simulink model "testbench_main2"  (R2016b)
settings: Solver=FixedStepAuto  StartTime=0.0  StopTime=inf  RelTol=1e-3  EnableMultiTasking=on
values from neighbouring files (symbols this model uses):
  b = 16    [Script_controller.m]
libraries: legoev3lib x4
settings Model: SimulationMode=external  ExtModeTrigDuration=2  Creator=Shobhit  LastModifiedBy=karanverma
settings SolverCC: PositivePriorityOrder=on
settings OptimizationCC: LifeSpan=1  MaxStackSize=64
settings DebuggingCC: SFUnexpectedBacktrackingDiag=warning  SFNoUnconditionalDefaultTransitionDiag=warning  SFExecutionAtInitializationDiag=none
settings HardwareCC: ProdBitPerPointer=32  ProdBitPerSizeT=32  ProdBitPerPtrDiffT=32  ProdLargestAtomicInteger=Long  ProdWordSize=32  ProdHWDeviceType=ARM Compatible->ARM 9  UseEmbeddedCoderFeatures=off  UseSimulinkCoderFeatures=off
settings RTWCC: SystemTargetFile=ert.tlc  HardwareBoard=LEGO MINDSTORMS EV3  TLCOptions=-aInlineSetEventsForThisBaseRateFcn=TLC_FALSE -aSuppressMultiTaskScheduler=TLC_FALSE -aRateBasedStepFcn=0  TemplateMakefile=ert_default_tmf  Description=Embedded Coder  GenerateReport=on  Toolchain=Sourcery G++ Lite v2009q3  LaunchReport=on
settings CodeAppCC: ForceParamTrailComments=on  OperatorAnnotations=on  MATLABSourceComments=on
settings ERTTargetCC: ERTCustomFileBanners=off  SupportContinuousTime=on  SupportNonInlinedSFcns=on  SupportVariableSizeSignals=on  ModelStepFunctionPrototypeControlCompliant=off
settings ConfigComp: CovMetricSettings=dw  CovHtmlReporting=on  CovSaveCumulativeToWorkspaceVar=on  CovSaveSingleToWorkspaceVar=on  CovExternalEMLEnable=off

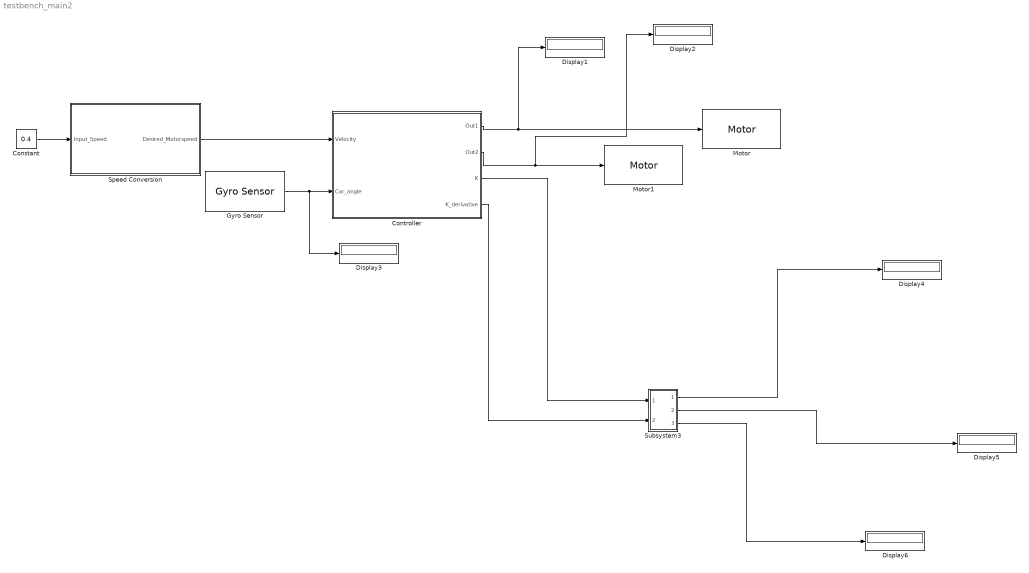
== system testbench_main2 ==
  Constant : Constant  Value=0.4
  Controller : Subsystem
  Display{1..6} (6 alike) : Display
      Display4 settings: Decimation=2
  Gyro Sensor : legoev3lib/Gyro Sensor  portNumber=1  sampleTime=0.1
  Motor : legoev3lib/Motor  sportNumber=A  sstopAction=Brake
  Motor1 : legoev3lib/Motor  sportNumber=B  sstopAction=Brake
  Speed Conversion : Subsystem
  Subsystem3 : Subsystem
  wires:
  Gyro Sensor/1 -> Display3/1, Controller/2(Car_angle)
  Constant/1 -> Speed Conversion/1(Input_Speed)
  Controller/1(Out1) -> Motor/1, Display1/1
  Controller/2(Out2) -> Display2/1, Motor1/1
  Speed Conversion/1(Desired_Motorspeed) -> Controller/1(Velocity)
  Controller/4(K_derivative) -> Subsystem3/2(In2)
  Subsystem3/1(Out1) -> Display4/1
  Subsystem3/2(Out2) -> Display5/1
  Subsystem3/3(Out3) -> Display6/1
  Controller/3(K) -> Subsystem3/1(In1)

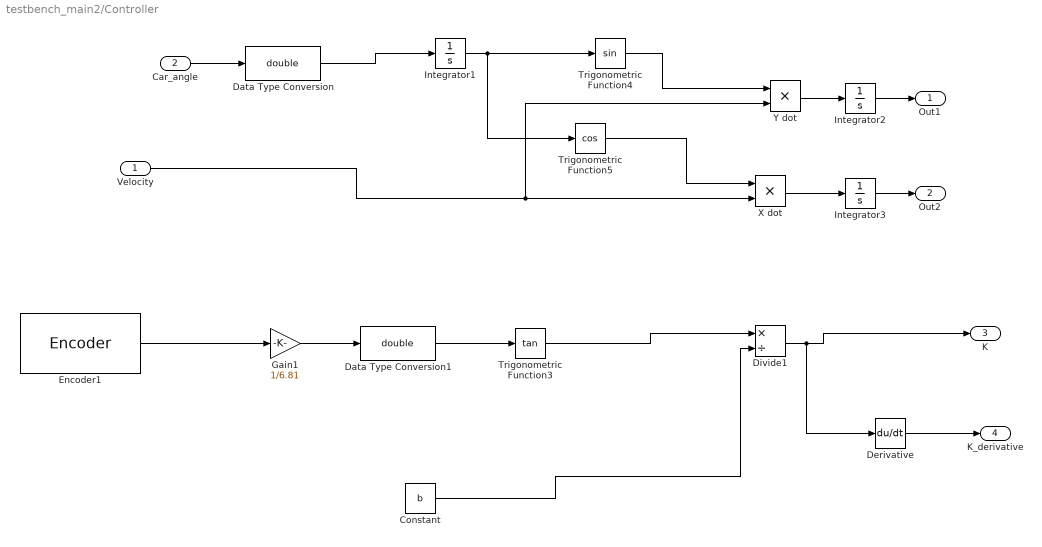
== system testbench_main2/Controller ==
  Velocity : Inport
  Car_angle : Inport  Port=2
  Constant : Constant  Value=b
  Data Type Conversion : DataTypeConversion  OutDataTypeStr=double
  Data Type Conversion1 : DataTypeConversion  OutDataTypeStr=double
  Derivative : Derivative
  Divide1 : Product  Inputs=*/
  Encoder1 : legoev3lib/Encoder  portNumber=A  opMode=No reset  sampleTime=0.1
  Gain1 : Gain  Gain=1/6.81
  Integrator1 : Integrator
  Integrator2 : Integrator
  Integrator3 : Integrator
  Trigonometric Function3 : Trigonometry  Operator=tan  OutputSignalType=real
  Trigonometric Function4 : Trigonometry
  Trigonometric Function5 : Trigonometry  Operator=cos
  "X dot " : Product
  "Y dot " : Product
  Out1 : Outport
  Out2 : Outport  Port=2
  K : Outport  Port=3
  K_derivative : Outport  Port=4
  wires:
  Car_angle/1 -> Data Type Conversion/1
  Encoder1/1 -> Gain1/1
  Gain1/1 -> Data Type Conversion1/1
  Constant/1 -> Divide1/2
  Integrator1/1 -> Trigonometric Function5/1, Trigonometric Function4/1
  Velocity/1 -> "Y dot "/2, "X dot "/2
  Trigonometric Function5/1 -> "X dot "/1
  Trigonometric Function4/1 -> "Y dot "/1
  "X dot "/1 -> Integrator3/1
  "Y dot "/1 -> Integrator2/1
  Data Type Conversion/1 -> Integrator1/1
  Integrator2/1 -> Out1/1
  Integrator3/1 -> Out2/1
  Divide1/1 -> Derivative/1, K/1
  Trigonometric Function3/1 -> Divide1/1
  Data Type Conversion1/1 -> Trigonometric Function3/1
  Derivative/1 -> K_derivative/1

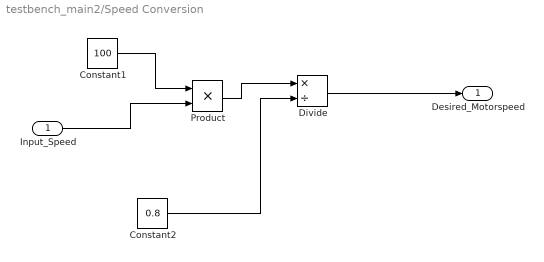
== system testbench_main2/Speed Conversion ==
  Input_Speed : Inport
  Constant1 : Constant  Value=100
  Constant2 : Constant  Value=0.8
  Divide : Product  Inputs=*/
  Product : Product
  Desired_Motorspeed : Outport
  wires:
  Divide/1 -> Desired_Motorspeed/1
  Input_Speed/1 -> Product/2
  Constant2/1 -> Divide/2
  Product/1 -> Divide/1
  Constant1/1 -> Product/1

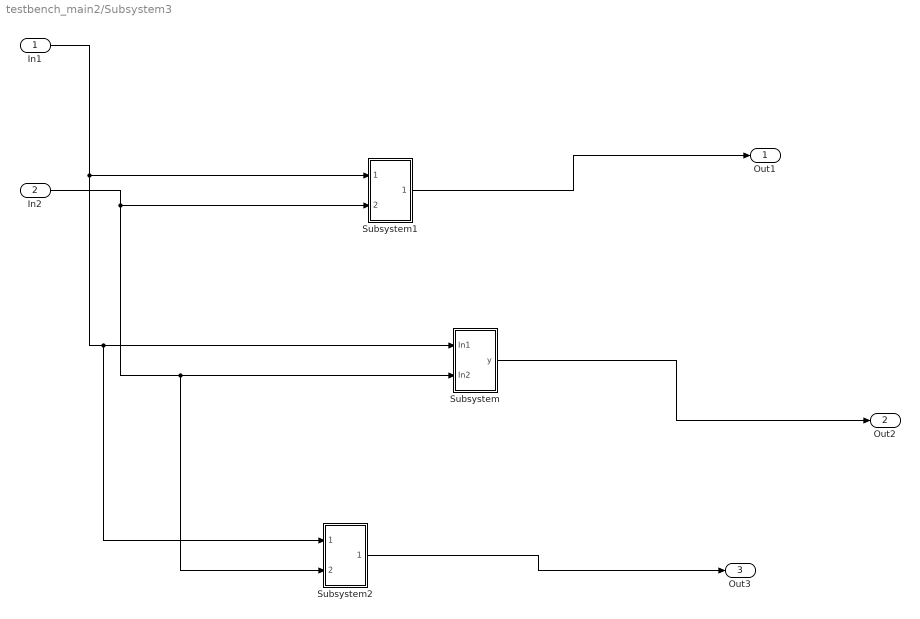
== system testbench_main2/Subsystem3 ==
  In1 : Inport
  In2 : Inport  Port=2
  Subsystem : Subsystem
  Subsystem1 : Subsystem
  Subsystem2 : Subsystem
  Out1 : Outport
  Out2 : Outport  Port=2
  Out3 : Outport  Port=3
  wires:
  Subsystem1/1(Out1) -> Out1/1
  Subsystem2/1(Out1) -> Out3/1
  In2/1 -> Subsystem1/2(In2), Subsystem2/2(In2), Subsystem/2(In2)
  Subsystem/1(y) -> Out2/1
  In1/1 -> Subsystem1/1(In1), Subsystem2/1(In1), Subsystem/1(In1)

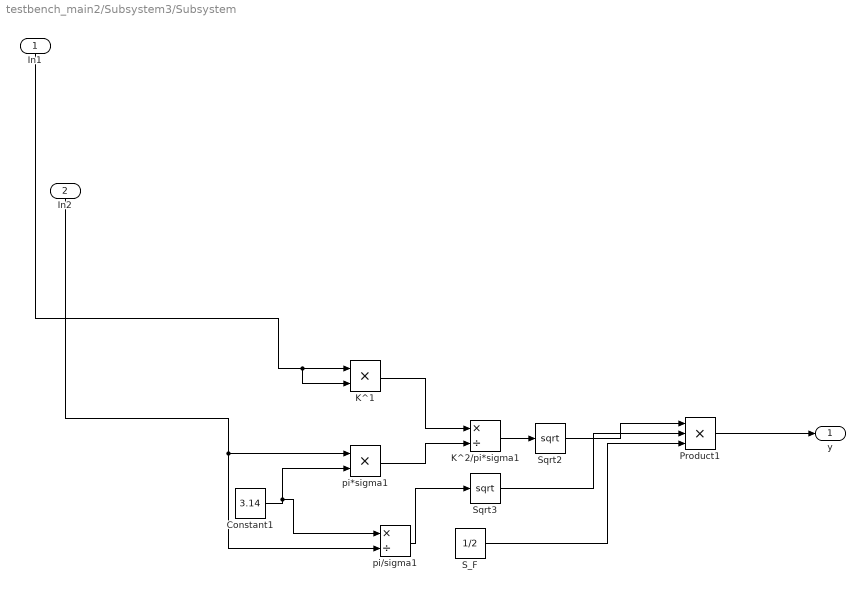
== system testbench_main2/Subsystem3/Subsystem ==
  In1 : Inport
  In2 : Inport  Port=2
  Constant1 : Constant  Value=3.14
  K^1 : Product
  K^2/pi*sigma1 : Product  Inputs=*/
  Product1 : Product  Inputs=3
  S_F : Constant  Value=1/2
  Sqrt2 : Sqrt  SaturateOnIntegerOverflow=on
  Sqrt3 : Sqrt  SaturateOnIntegerOverflow=on
  pi*sigma1 : Product
  pi/sigma1 : Product  Inputs=*/
  y : Outport
  wires:
  Constant1/1 -> pi/sigma1/1, pi*sigma1/2
  K^1/1 -> K^2/pi*sigma1/1
  pi*sigma1/1 -> K^2/pi*sigma1/2
  K^2/pi*sigma1/1 -> Sqrt2/1
  Sqrt2/1 -> Product1/1
  pi/sigma1/1 -> Sqrt3/1
  S_F/1 -> Product1/3
  Sqrt3/1 -> Product1/2
  Product1/1 -> y/1
  In2/1 -> pi/sigma1/2, pi*sigma1/1
  In1/1 -> K^1/2, K^1/1

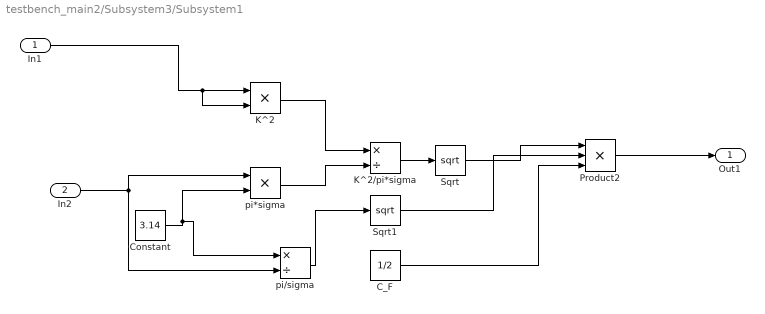
== system testbench_main2/Subsystem3/Subsystem1 ==
  In1 : Inport
  In2 : Inport  Port=2
  C_F : Constant  Value=1/2
  Constant : Constant  Value=3.14
  K^2 : Product
  K^2/pi*sigma : Product  Inputs=*/
  Product2 : Product  Inputs=3
  Sqrt : Sqrt  SaturateOnIntegerOverflow=on
  Sqrt1 : Sqrt  SaturateOnIntegerOverflow=on
  pi*sigma : Product
  pi/sigma : Product  Inputs=*/
  Out1 : Outport
  wires:
  Sqrt1/1 -> Product2/2
  pi*sigma/1 -> K^2/pi*sigma/2
  Product2/1 -> Out1/1
  Constant/1 -> pi/sigma/1, pi*sigma/2
  In2/1 -> pi*sigma/1, pi/sigma/2
  In1/1 -> K^2/2, K^2/1
  K^2/1 -> K^2/pi*sigma/1
  Sqrt/1 -> Product2/1
  pi/sigma/1 -> Sqrt1/1
  C_F/1 -> Product2/3
  K^2/pi*sigma/1 -> Sqrt/1

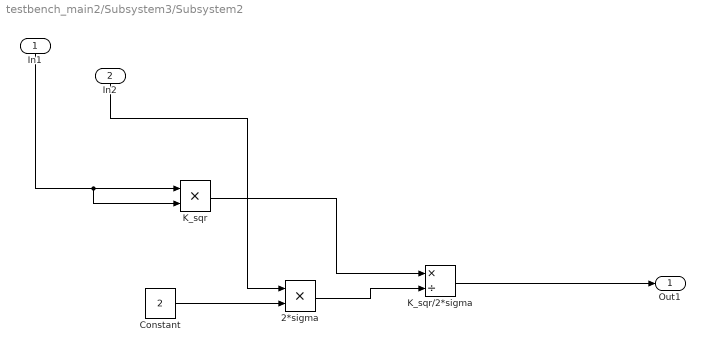
== system testbench_main2/Subsystem3/Subsystem2 ==
  In1 : Inport
  In2 : Inport  Port=2
  2*sigma : Product
  Constant : Constant  Value=2
  K_sqr : Product
  K_sqr/2*sigma : Product  Inputs=*/
  Out1 : Outport
  wires:
  In2/1 -> 2*sigma/1
  In1/1 -> K_sqr/2, K_sqr/1
  Constant/1 -> 2*sigma/2
  K_sqr/2*sigma/1 -> Out1/1
  2*sigma/1 -> K_sqr/2*sigma/2
  K_sqr/1 -> K_sqr/2*sigma/1
